simulink model "ep4_5"  (R2023b)
settings: Solver=VariableStepAuto  StartTime=0.0  StopTime=20  MaxStep=0.1  RelTol=1e-6
settings Model: Creator=86186  LastModifiedBy=86186

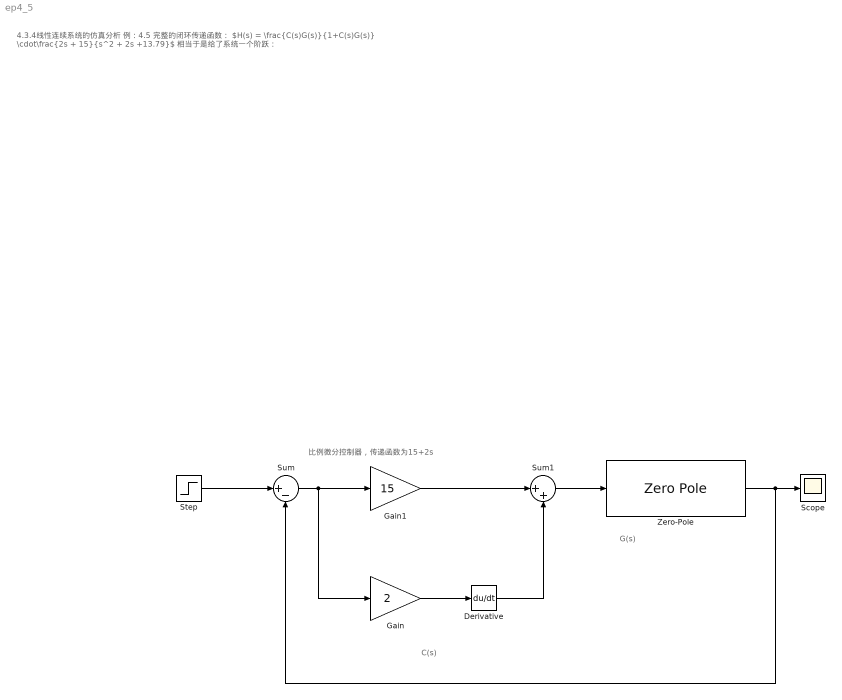
== system ep4_5 ==
  note: C(s)
  note: 比例微分控制器，传递函数为15+2s
  note: 4.3.4线性连续系统的仿真分析
      | 例：4.5
      | 完整的闭环传递函数：
      | $H(s) = \frac{C(s)G(s)}{1+C(s)G(s)} \cdot\frac{2s + 15}{s^2 + 2s +13.79}$
      |
      | 相当于是给了系统一个阶跃：
  note: G(s)
  Derivative : Derivative
  Gain : Gain  Gain=2
  Gain1 : Gain  Gain=15
  Scope : Scope
  Step : Step  SampleTime=0
  Sum : Sum  Inputs=|+-
  Sum1 : Sum  Inputs=|++
  Zero-Pole : ZeroPole  Zeros=[]  Poles=[1.1 -1.1]
  wires:
  Sum/1 -> Gain/1, Gain1/1
  Gain1/1 -> Sum1/1
  Gain/1 -> Derivative/1
  Derivative/1 -> Sum1/2
  Sum1/1 -> Zero-Pole/1
  Zero-Pole/1 -> Sum/2, Scope/1
  Step/1 -> Sum/1
